simulink model "TischMal2"  (Simulink 7.9)
settings: Solver=ode45  StartTime=0.0  StopTime=10  MaxStep=0.1  RelTol=1e-3
settings Model: Creator=karo  LastModifiedBy=karo

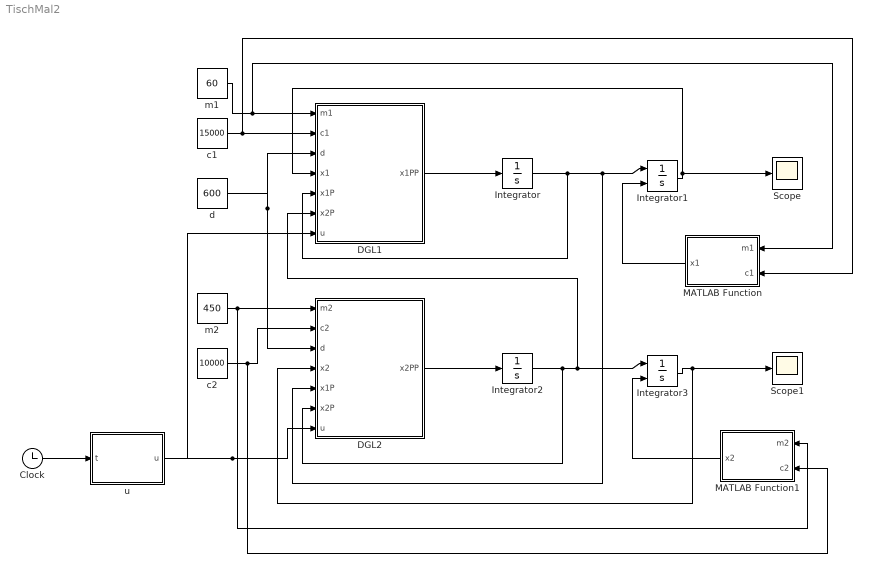
== system TischMal2 ==
  Clock : Clock
  DGL1 : MATLAB Function  TreatAsAtomicUnit=on
  DGL2 : MATLAB Function  TreatAsAtomicUnit=on
  Integrator : Integrator
  Integrator1 : Integrator  InitialConditionSource=external
  Integrator2 : Integrator
  Integrator3 : Integrator  InitialConditionSource=external
  MATLAB Function : MATLAB Function  TreatAsAtomicUnit=on
  MATLAB Function1 : MATLAB Function  TreatAsAtomicUnit=on
  Scope : Scope
  Scope1 : Scope
  c1 : Constant  Value=15000
  c2 : Constant  Value=10000
  d : Constant  Value=600
  m1 : Constant  Value=60
  m2 : Constant  Value=450
  u : MATLAB Function  TreatAsAtomicUnit=on
  wires:
  m1/1 -> DGL1/1(m1), MATLAB Function/1(m1)
  c1/1 -> DGL1/2(c1), MATLAB Function/2(c1)
  DGL1/1(x1PP) -> Integrator/1
  Integrator/1 -> DGL1/5(x1P), Integrator1/1, DGL2/5(x1P)
  d/1 -> DGL1/3(d), DGL2/3(d)
  m2/1 -> DGL2/1(m2), MATLAB Function1/1(m2)
  c2/1 -> DGL2/2(c2), MATLAB Function1/2(c2)
  DGL2/1(x2PP) -> Integrator2/1
  Integrator2/1 -> DGL2/6(x2P), Integrator3/1, DGL1/6(x2P)
  Integrator1/1 -> DGL1/4(x1), Scope/1
  Integrator3/1 -> DGL2/4(x2), Scope1/1
  Clock/1 -> u/1(t)
  u/1(u) -> DGL2/7(u), DGL1/7(u)
  MATLAB Function/1(x1) -> Integrator1/2
  MATLAB Function1/1(x2) -> Integrator3/2

== matlab function DGL2 ==
  data: m2 input double; c2 input double; d input double; x2 input double; x1P input double; x2P input double; u input double; x2PP output double
function x2PP = fcn(m2, c2, d, x2, x1P, x2P, u)
%#codegen

g = -9.81;   % Gravitationskonstante

%x2PP = (-m2*g - c2*(x2 - u) - d*(x2P - x1P)) / m2;
x2PP = (2*(-c2 * (x2 - u)) + 2*(-d*(x2P - x1P)) + (m2*g)) / m2;

== matlab function DGL1 ==
  data: m1 input double; c1 input double; d input double; x1 input double; x1P input double; x2P input double; u input double; x1PP output double
function x1PP = fcn(m1, c1, d, x1, x1P, x2P, u)
%#codegen

g = -9.81;   % Gravitationskonstante
x1PP = (2*(-c1 * (x1 - u)) + 2*(d*(x2P - x1P)) + (m1*g)) / m1;
%x1PP = (-m1*g - c1*(x1 - u) + d*(x2P - x1P)) / m1;

== matlab function u ==
  data: u output double; t input double
function u = fcn(t)
%#codegen
if (t <= 1)
    u = 0;
else
    u = 0.001;
end

== matlab function MATLAB Function ==
  data: m1 input double; x1 output double; c1 input double
function x1 = fcn(m1, c1)

g = -9.81;

x1 = (m1*g) / (2*c1);

== matlab function MATLAB Function1 ==
  data: m2 input double; x2 output double; c2 input double
function x2 = fcn(m2, c2)

g = -9.81;

x2 = (m2*g) / (2*c2);
